simulink model "LQI_solar_2017a"  (Simulink 8.9)
settings: Solver=VariableStepAuto  StartTime=0.0  StopTime=100000  FixedStep=1  RelTol=1e-1
values from neighbouring files (symbols this model uses):
  A_solar_tank_1 = eval(A_solar_tank)    [solar_tank_lqi_init.m]
  B_solar_tank_1 = eval(B_solar_tank(:,1:2))    [solar_tank_lqi_init.m]
  Bd_solar_tank_1 = eval(B_solar_tank(:,3:5))    [solar_tank_lqi_init.m]
  C_solar_tank_1 = eye(3)    [solar_tank_lqi_init.m]
  Ki = lqr(Ai, Bi, Qi, Ri)    [solar_tank_lqi_init.m]
settings Model: Creator=admin  LastModifiedBy=admin
settings DataIOCC: LimitDataPoints=off  SaveFormat=Dataset  SignalLoggingSaveFormat=Dataset
settings OptimizationCC: LifeSpan=auto
settings DebuggingCC: UnderspecifiedInitializationDetection=Simplified  MergeDetectMultiDrivingBlocksExec=error  FcnCallInpInsideContextMsg=error  StateNameClashWarn=none  SFUnexpectedBacktrackingDiag=error  SFNoUnconditionalDefaultTransitionDiag=error  SFExecutionAtInitializationDiag=warning
settings HardwareCC: ProdBitPerPointer=64  ProdBitPerSizeT=64  ProdBitPerPtrDiffT=64  ProdLargestAtomicFloat=Float  ProdIntDivRoundTo=Zero  ProdEndianess=LittleEndian  ProdWordSize=64  ProdHWDeviceType=Intel->x86-64 (Windows64)
settings ModelReferenceCC: PropagateSignalLabelsOutOfModel=on
settings GRTTargetCC: TargetLangStandard=C99 (ISO)  GeneratePreprocessorConditionals=Use local settings  CombineOutputUpdateFcns=on  GRTInterface=off
settings ConfigComp: CovMetricSettings=dwe  CovHtmlReporting=off  CovSaveCumulativeToWorkspaceVar=off  CovSaveSingleToWorkspaceVar=off  CovExternalEMLEnable=on

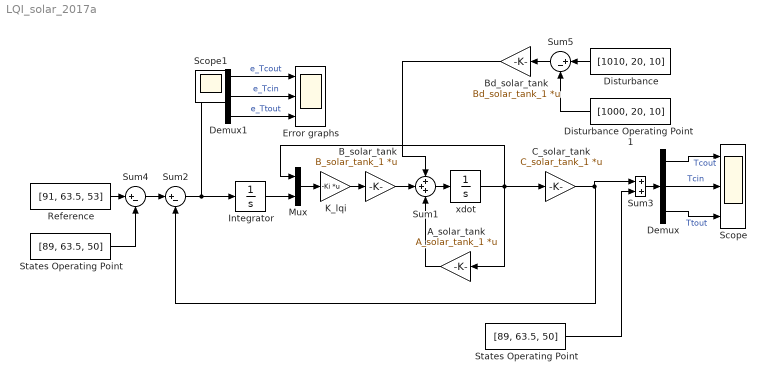
== system LQI_solar_2017a ==
  A_solar_tank : Gain  Gain=A_solar_tank_1  Multiplication=Matrix(K*u)
  B_solar_tank : Gain  Gain=B_solar_tank_1  Multiplication=Matrix(K*u)
  Bd_solar_tank : Gain  Gain=Bd_solar_tank_1  Multiplication=Matrix(K*u)
  C_solar_tank : Gain  Gain=C_solar_tank_1  Multiplication=Matrix(K*u)
  Demux : Demux  Outputs=3
  Demux1 : Demux  Outputs=3
  Disturbance : Constant  Value=[1010, 20, 10]
  Disturbance Operating Point   1 : Constant  Value=[1000, 20, 10]
  Error graphs : Scope  NumInputPorts=3
  Integrator : Integrator  InitialCondition=[0;0;0]
  K_lqi : Gain  Gain=-Ki  Multiplication=Matrix(K*u)
  Mux : Mux  Inputs=2
  Reference : Constant  Value=[91, 63.5, 53]
  Scope : Scope  NumInputPorts=3
  "States Operating Point " : Constant  Value=[89, 63.5, 50]
  "States Operating Point   " : Constant  Value=[89, 63.5, 50]
  Sum1 : Sum  Inputs=+++
  Sum2 : Sum  Inputs=|+-
  Sum3 : Sum
  Sum4 : Sum  Inputs=|+-
  Sum5 : Sum  Inputs=|+-
  xdot : Integrator  InitialCondition=[0;0;0]
  Scope1 : Scope
  wires:
  Sum2/1 -> Demux1/1, Integrator/1
  Integrator/1 -> Mux/2
  K_lqi/1 -> B_solar_tank/1
  Sum1/1 -> xdot/1
  C_solar_tank/1 -> Sum3/1, Sum2/2
  Mux/1 -> K_lqi/1
  xdot/1 -> A_solar_tank/1, C_solar_tank/1, Mux/1
  Demux/1 -> Scope/1  "Tcout"
  Demux/2 -> Scope/2  "Tcin"
  Demux/3 -> Scope/3  "Ttout"
  Demux1/2 -> Error graphs/2  "e_Tcin"
  Demux1/1 -> Error graphs/1  "e_Tcout"
  Demux1/3 -> Error graphs/3  "e_Ttout"
  Sum5/1 -> Bd_solar_tank/1
  A_solar_tank/1 -> Sum1/3
  B_solar_tank/1 -> Sum1/2
  Bd_solar_tank/1 -> Sum1/1
  Sum3/1 -> Demux/1
  "States Operating Point "/1 -> Sum3/2
  Reference/1 -> Sum4/1
  Sum4/1 -> Sum2/1
  "States Operating Point   "/1 -> Sum4/2
  Disturbance Operating Point   1/1 -> Sum5/2
  Disturbance/1 -> Sum5/1
